simulink model "verify_PipeBasicNodes_mdl"  (R2016b)
settings: Solver=ode45  StartTime=0.0  StopTime=2*3600  RelTol=1e-3  EnableMultiTasking=on
libraries: carnot x3, simulink x1
settings Model: Creator=drhf  LastModifiedBy=drhf
settings DataIOCC: LimitDataPoints=on  SaveFormat=Array  SignalLoggingSaveFormat=ModelDataLogs  SignalLogging=off
settings OptimizationCC: ExpressionDepthLimit=2147483647  LifeSpan=inf
settings DebuggingCC: UnderspecifiedInitializationDetection=Classic  MergeDetectMultiDrivingBlocksExec=none  SolverPrmCheckMsg=warning  FcnCallInpInsideContextMsg=warning  StateNameClashWarn=warning  SFUnexpectedBacktrackingDiag=warning  SFNoUnconditionalDefaultTransitionDiag=warning  SFExecutionAtInitializationDiag=none
settings HardwareCC: ProdBitPerPointer=32  ProdBitPerSizeT=32  ProdBitPerPtrDiffT=32  ProdLargestAtomicFloat=None  ProdIntDivRoundTo=Undefined  ProdEndianess=Unspecified  ProdWordSize=32  ProdHWDeviceType=32-bit Generic
settings ModelReferenceCC: PropagateSignalLabelsOutOfModel=off
settings GRTTargetCC: TargetLangStandard=C89/C90 (ANSI)  GeneratePreprocessorConditionals=Disable all  CombineOutputUpdateFcns=off  GRTInterface=on
settings ConfigComp: CovMetricSettings=dw  CovHtmlReporting=on  CovSaveCumulativeToWorkspaceVar=on  CovSaveSingleToWorkspaceVar=on  CovExternalEMLEnable=off

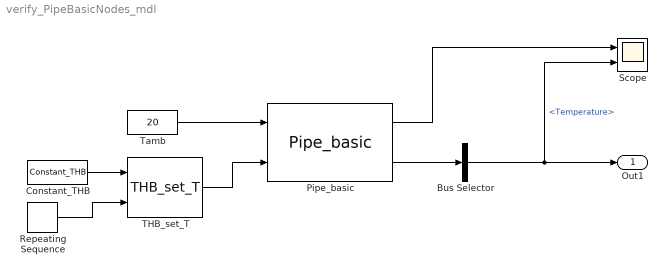
== system verify_PipeBasicNodes_mdl ==
  Bus Selector : BusSelector  OutputSignals=Temperature
  Constant_THB : carnot/Source/Simple/Constant_THB  t=40  mdot=30/3600  p=1e5  mID=No Pressure Drop  fluid=Water  mix=0  mix2=0  mix3=0  dia=0.02  hgt=0
  Pipe_basic : carnot/Basic/Thermal_Models/Pipe_basic  vol="sqrt(0.01/(10*pi))      % 10 liter on 10 m"  L=10  uloss=0  effcond=0  cwall=0  t0=20  nodes=1
  Repeating Sequence : simulink/Sources/Repeating Sequence  rep_seq_t=[0 0.5 0.501 2.01]*3600  rep_seq_y=[60 60 20 20]
  Scope : Scope  NumInputPorts=2
  THB_set_T : carnot/Source/Simple/THB_set_T
  Tamb : Constant  Value=20
  Out1 : Outport  SampleTime=60
  wires:
  Tamb/1 -> Pipe_basic/1
  THB_set_T/1 -> Pipe_basic/2
  Pipe_basic/2 -> Bus Selector/1
  Pipe_basic/1 -> Scope/1
  Constant_THB/1 -> THB_set_T/1
  Repeating Sequence/1 -> THB_set_T/2
  Bus Selector/1 -> Scope/2, Out1/1  "<Temperature>"
